simulink model "flightControlSystem"  (R2024a)
settings: Solver=ode3  StartTime=0  StopTime=TFinal  FixedStep=Ts  RelTol=1e-3  EnableMultiTasking=on
undefined symbols (not defined in the file or in its folder): BINARIZER_THRESHOLD, codertarget, COG_X, COG_Y, Controller, DiscIntNeverNeededParam, Discrete, DISK_KERNEL, Estimator, FLAG_WAIT_FOR_HOVERING, FOV, FRAME_SIZE_HEIGHT, FRAME_SIZE_WIDTH, g, G_B_GAIN, gray, init, MAX_RADIUS_CROWN, MIN_RADIUS_CROWN, orient_ref, pos_ref, Sensors, SQUARE_KERNEL, strel, Time, Ts, Vehicle, Z_HIGH, Z_LOW
libraries: simulink x35, sharedtransform x3, ctrlSharedLib x2, visionmorphops x2, sharedutil x1, parrotlib x1
(part 2 of 2)

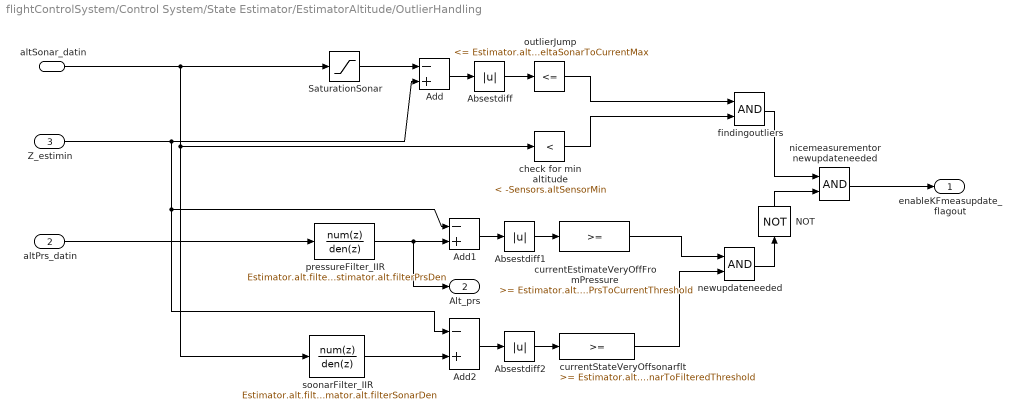
== system flightControlSystem/Control System/State Estimator/EstimatorAltitude/OutlierHandling ==
  altSonar_datin : Inport
  altPrs_datin : Inport  Port=2
  Z_estimin : Inport  Port=3
  Absestdiff : Abs  SaturateOnIntegerOverflow=off
  Absestdiff1 : Abs  SaturateOnIntegerOverflow=off
  Absestdiff2 : Abs  SaturateOnIntegerOverflow=off
  Add : Sum  Inputs=-+
  Add1 : Sum  Inputs=-+
  Add2 : Sum  Inputs=-+
  NOT : Logic  Operator=NOT  IconShape=distinctive  AllPortsSameDT=off  OutDataTypeStr=boolean
  SaturationSonar : Saturate  UpperLimit=-Sensors.altSensorMin  LowerLimit=-inf
  check for min altitude : simulink/Logic and Bit Operations/Compare To Constant  relop=<  const=-Sensors.altSensorMin  OutDataTypeStr=boolean
  currentEstimateVeryOffFromPressure : simulink/Logic and Bit Operations/Compare To Constant  relop=>=  const=Estimator.alt.deltaPrsToCurrentThreshold  OutDataTypeStr=boolean
  currentStateVeryOffsonarflt : simulink/Logic and Bit Operations/Compare To Constant  relop=>=  const=Estimator.alt.deltaSonarToFilteredThreshold  OutDataTypeStr=boolean
  findingoutliers : Logic  AllPortsSameDT=off  OutDataTypeStr=boolean
  newupdateneeded : Logic  AllPortsSameDT=off  OutDataTypeStr=boolean
  nicemeasurementor newupdateneeded : Logic  AllPortsSameDT=off  OutDataTypeStr=boolean
  outlierJump : simulink/Logic and Bit Operations/Compare To Constant  relop=<=  const=Estimator.alt.deltaSonarToCurrentMax  OutDataTypeStr=boolean
  pressureFilter_IIR : DiscreteFilter  Numerator=Estimator.alt.filterPrsNum  Denominator=Estimator.alt.filterPrsDen
  soonarFilter_IIR : DiscreteFilter  Numerator=Estimator.alt.filterSonarNum  Denominator=Estimator.alt.filterSonarDen
  enableKFmeasupdate_flagout : Outport  VectorParamsAs1DForOutWhenUnconnected=off
  Alt_prs : Outport  Port=2  VectorParamsAs1DForOutWhenUnconnected=off
  wires:
  Add1/1 -> Absestdiff1/1
  nicemeasurementor newupdateneeded/1 -> enableKFmeasupdate_flagout/1
  findingoutliers/1 -> nicemeasurementor newupdateneeded/1
  check for min altitude/1 -> findingoutliers/2
  outlierJump/1 -> findingoutliers/1
  SaturationSonar/1 -> Add/1
  Absestdiff/1 -> outlierJump/1
  Add/1 -> Absestdiff/1
  newupdateneeded/1 -> NOT/1
  Absestdiff2/1 -> currentStateVeryOffsonarflt/1
  altSonar_datin/1 -> SaturationSonar/1, soonarFilter_IIR/1, check for min altitude/1
  currentEstimateVeryOffFromPressure/1 -> newupdateneeded/1
  Z_estimin/1 -> Add1/1, Add2/1, Add/2
  Add2/1 -> Absestdiff2/1
  currentStateVeryOffsonarflt/1 -> newupdateneeded/2
  pressureFilter_IIR/1 -> Alt_prs/1, Add1/2
  altPrs_datin/1 -> pressureFilter_IIR/1
  soonarFilter_IIR/1 -> Add2/2
  Absestdiff1/1 -> currentEstimateVeryOffFromPressure/1
  NOT/1 -> nicemeasurementor newupdateneeded/2

== system flightControlSystem/Control System/State Estimator/EstimatorXYPosition/EstimatorVelocity ==
  opticalFlow_datin : Inport
  Z_estimin : Inport  Port=2  SampleTime=Ts
  sensorIMU_datin : Inport  Port=3
  orient_estimin : Inport  Port=4
  " " : Product  Inputs=**
  AccelerationHandling : Subsystem
  Compare To Constant : simulink/Logic and Bit Operations/Compare To Constant  relop=<  const=200*4  OutDataTypeStr=boolean
  Counter Free-Running : simulink/Sources/Counter Free-Running  NumBits=32  tsamp=-1
  DataHandling : Subsystem
  Delay : Delay  DelayLength=1  InitialCondition=0
  Gain : Gain  Gain=-1
  KalmanFilter_dxdy : ctrlSharedLib/Kalman Filter  TimeDomain=Discrete-Time  UseCurrentEstimator=on  ModelSource=Individual A, B, C, D matrices  ModelSourceVariable=ss(0.95,1,1,0,1)  A=eye(2)  B=Ts*eye(2)  C=eye(2)  D=0  NumberOfStates=1  NumberOfInputs=1  NumberOfOutputs=1  InitialEstimateSource=Dialog  X0=0  P0=10  UseK=off  UseGH=on  NumberOfProcessNoiseInputs=1  G=Estimator.pos.kfVelo.G  TimeInvariantG=on  H=Estimator.pos.kfVelo.H  TimeInvariantH=on  Q=Estimator.pos.kfVelo.Q  TimeInvariantQ=on  R=Estimator.pos.kfVelo.R  TimeInvariantR=on  N=Estimator.pos.kfVelo.N  TimeInvariantN=on  AddInputPort=on  AddEnablePort=on  OutputEstimatedY=off  OutputP=off  Ts=-1
  Select dxy : Selector  InputPortWidth=3  IndexOptions=Index vector (dialog)  Indices=[1 2]  OutputSizes=1
  Switch : Switch  Criteria=u2 > Threshold  SaturateOnIntegerOverflow=off  InputSameDT=off
  Z_estimin1 : InportShadow  Port=2  SampleTime=Ts
  opticalFlowErrorCorrect : Gain  Gain=1.15
  dxy_estimout : Outport  VectorParamsAs1DForOutWhenUnconnected=off
  wires:
  Delay/1 -> DataHandling/5(dxyOF_datin)
  Z_estimin/1 -> DataHandling/1(Z_estimin), AccelerationHandling/4(Z_estimin)
  KalmanFilter_dxdy/1 -> dxy_estimout/1, Delay/1
  sensorIMU_datin/1 -> AccelerationHandling/2(sensorIMU_datin), DataHandling/3(sensorIMU_datin)
  orient_estimin/1 -> AccelerationHandling/3(orient_estimin), DataHandling/2(orient_estimin)
  Select dxy/1 -> KalmanFilter_dxdy/2, AccelerationHandling/1(dxy_estimin), DataHandling/4(dxy_estimin)
  AccelerationHandling/1(acceleration_world) -> KalmanFilter_dxdy/1
  DataHandling/1(enable_flag) -> KalmanFilter_dxdy/3
  Switch/1 -> Select dxy/1
  " "/1 -> opticalFlowErrorCorrect/1
  Gain/1 -> " "/2
  opticalFlowErrorCorrect/1 -> Switch/3
  Compare To Constant/1 -> Switch/2
  opticalFlow_datin/1 -> " "/1, Switch/1
  Z_estimin1/1 -> Gain/1
  Counter Free-Running/1 -> Compare To Constant/1

== system flightControlSystem/Control System/State Estimator/EstimatorXYPosition/EstimatorXYPosition ==
  note: Switching from orientationControl to Position
      | control reset the current world position estimate
      | (happens when using no markers)
  dxy_estimin : Inport
  orient_estimin : Inport  Port=2  SampleTime=Ts
  controlModePosVSOrient_flagin : Inport  Port=3
  dz_estimin : Inport  Port=4
  Math Function : Math  Operator=transpose  SignedPower=on
  Mux2 : Mux  Inputs=2
  Product : Product  Multiplication=Matrix(*)
  Rotation Angles to Direction Cosine Matrix : sharedtransform/Rotation Angles to Direction Cosine Matrix  rotationOrder=ZYX  aMode=aMode
  SelectdXY : Selector  InputPortWidth=3  IndexOptions=Index vector (dialog)  Indices=[1 2]  OutputSizes=1
  SimplyIntegrateVelocity : DiscreteIntegrator  ExternalReset=rising  SampleTime=Ts  ICPrevOutput=DiscIntNeverNeededParam  ICPrevScaledInput=DiscIntNeverNeededParam
  XY_estimout : Outport  VectorParamsAs1DForOutWhenUnconnected=off
  wires:
  controlModePosVSOrient_flagin/1 -> SimplyIntegrateVelocity/2
  Product/1 -> SelectdXY/1
  Mux2/1 -> Product/2
  dz_estimin/1 -> Mux2/2
  SimplyIntegrateVelocity/1 -> XY_estimout/1
  dxy_estimin/1 -> Mux2/1
  orient_estimin/1 -> Rotation Angles to Direction Cosine Matrix/1
  Rotation Angles to Direction Cosine Matrix/1 -> Math Function/1
  SelectdXY/1 -> SimplyIntegrateVelocity/1
  Math Function/1 -> Product/1

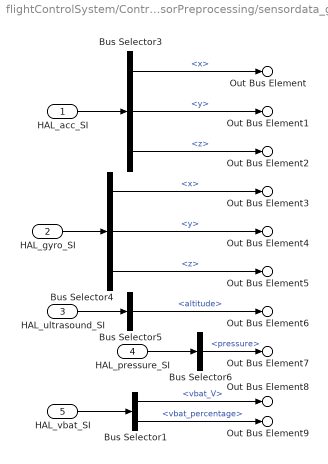
== system flightControlSystem/Control System/State Estimator/SensorPreprocessing/sensordata_group ==
  HAL_acc_SI : Inport  OutDataTypeStr=Bus: HAL_acc_SI_t
  HAL_gyro_SI : Inport  Port=2  OutDataTypeStr=Bus: HAL_gyro_SI_t
  HAL_ultrasound_SI : Inport  Port=3  OutDataTypeStr=Bus: HAL_ultrasound_SI_t
  HAL_pressure_SI : Inport  Port=4  OutDataTypeStr=Bus: HAL_pressure_SI_t
  HAL_vbat_SI : Inport  Port=5  OutDataTypeStr=Bus: HAL_vbat_SI_t
  Bus Selector1 : BusSelector  OutputSignals=vbat_V,vbat_percentage
  Bus Selector3 : BusSelector  OutputSignals=x,y,z
  Bus Selector4 : BusSelector  OutputSignals=x,y,z
  Bus Selector5 : BusSelector  OutputSignals=altitude
  Bus Selector6 : BusSelector  OutputSignals=pressure
  Out Bus Element : Outport  VectorParamsAs1DForOutWhenUnconnected=off  PortName=sensordata_datin  Element=ddx
  Out Bus Element1 : Outport  VectorParamsAs1DForOutWhenUnconnected=off  PortName=sensordata_datin  Element=ddy
  Out Bus Element2 : Outport  VectorParamsAs1DForOutWhenUnconnected=off  PortName=sensordata_datin  Element=ddz
  Out Bus Element3 : Outport  VectorParamsAs1DForOutWhenUnconnected=off  PortName=sensordata_datin  Element=p
  Out Bus Element4 : Outport  VectorParamsAs1DForOutWhenUnconnected=off  PortName=sensordata_datin  Element=q
  Out Bus Element5 : Outport  VectorParamsAs1DForOutWhenUnconnected=off  PortName=sensordata_datin  Element=r
  Out Bus Element6 : Outport  VectorParamsAs1DForOutWhenUnconnected=off  PortName=sensordata_datin  Element=altitude_sonar
  Out Bus Element7 : Outport  VectorParamsAs1DForOutWhenUnconnected=off  PortName=sensordata_datin  Element=prs
  Out Bus Element8 : Outport  VectorParamsAs1DForOutWhenUnconnected=off  PortName=sensordata_datin  Element=vbat_V
  Out Bus Element9 : Outport  VectorParamsAs1DForOutWhenUnconnected=off  PortName=sensordata_datin  Element=vbat_percentage
  wires:
  HAL_gyro_SI/1 -> Bus Selector4/1
  HAL_acc_SI/1 -> Bus Selector3/1
  HAL_pressure_SI/1 -> Bus Selector6/1
  HAL_ultrasound_SI/1 -> Bus Selector5/1
  Bus Selector4/1 -> Out Bus Element3/1  "<x>"
  Bus Selector3/3 -> Out Bus Element2/1  "<z>"
  Bus Selector4/3 -> Out Bus Element5/1  "<z>"
  Bus Selector5/1 -> Out Bus Element6/1  "<altitude>"
  Bus Selector6/1 -> Out Bus Element7/1  "<pressure>"
  Bus Selector4/2 -> Out Bus Element4/1  "<y>"
  Bus Selector3/1 -> Out Bus Element/1  "<x>"
  Bus Selector3/2 -> Out Bus Element1/1  "<y>"
  Bus Selector1/1 -> Out Bus Element8/1  "<vbat_V>"
  HAL_vbat_SI/1 -> Bus Selector1/1
  Bus Selector1/2 -> Out Bus Element9/1  "<vbat_percentage>"

== system flightControlSystem/Control System/State Estimator/EstimatorXYPosition/EstimatorVelocity/AccelerationHandling ==
  dxy_estimin : Inport
  sensorIMU_datin : Inport  Port=2
  orient_estimin : Inport  Port=3
  Z_estimin : Inport  Port=4
  Add : Sum  Inputs=-+
  Bus Selector1 : BusSelector  OutputSignals=ddx,ddy,ddz
  Deactivate Acceleration If OF is not used due to low altitude : simulink/Logic and Bit Operations/Compare To Constant  relop=<=  const=Estimator.pos.opticalFlowZMax  OutDataTypeStr=boolean
  Logical Operator : Logic  Operator=OR  AllPortsSameDT=off  OutDataTypeStr=boolean
  Mux6 : Mux  Inputs=3
  Product : Product  Inputs=3
  Product1 : Product  Multiplication=Matrix(*)
  Rotation Angles to Direction Cosine Matrix : sharedtransform/Rotation Angles to Direction Cosine Matrix  rotationOrder=ZYX  aMode=aMode
  SelectPlanarddxy : Selector  InputPortWidth=3  IndexOptions=Index vector (dialog)  Indices=[1 2]  OutputSizes=1
  Selector : Selector  InputPortWidth=2  IndexOptions=Index vector (dialog)  Indices=1  OutputSizes=1
  Selector1 : Selector  InputPortWidth=2  IndexOptions=Index vector (dialog)  Indices=2  OutputSizes=1
  do not use acc if optical flow never available (Note OF@60Hz but ZOH to 200!) : simulink/Logic and Bit Operations/Compare To Constant  relop=~=  const=0  OutDataTypeStr=boolean
  do not use acc if optical flow never available (Note OF@60Hz but ZOH to 200!)1 : simulink/Logic and Bit Operations/Compare To Constant  relop=~=  const=0  OutDataTypeStr=boolean
  gainaccinput : Gain  Gain=Estimator.pos.accelerationInputGain  OutDataTypeStr=single
  gravity : Constant  Value=[0 0 -g]
  acceleration_world : Outport  OutDataTypeStr=single  VectorParamsAs1DForOutWhenUnconnected=off
  wires:
  do not use acc if optical flow never available (Note OF@60Hz but ZOH to 200!)1/1 -> Logical Operator/2
  do not use acc if optical flow never available (Note OF@60Hz but ZOH to 200!)/1 -> Logical Operator/1
  Logical Operator/1 -> Product/1
  Selector1/1 -> do not use acc if optical flow never available (Note OF@60Hz but ZOH to 200!)1/1
  Selector/1 -> do not use acc if optical flow never available (Note OF@60Hz but ZOH to 200!)/1
  dxy_estimin/1 -> Selector1/1, Selector/1
  Product/1 -> acceleration_world/1
  Deactivate Acceleration If OF is not used due to low altitude/1 -> Product/3
  Z_estimin/1 -> Deactivate Acceleration If OF is not used due to low altitude/1
  Add/1 -> SelectPlanarddxy/1
  Product1/1 -> Add/1
  gravity/1 -> Product1/2
  gainaccinput/1 -> Product/2
  SelectPlanarddxy/1 -> gainaccinput/1
  Bus Selector1/3 -> Mux6/3  "<ddz>"
  Bus Selector1/1 -> Mux6/1  "<ddx>"
  sensorIMU_datin/1 -> Bus Selector1/1
  Mux6/1 -> Add/2
  Bus Selector1/2 -> Mux6/2  "<ddy>"
  orient_estimin/1 -> Rotation Angles to Direction Cosine Matrix/1
  Rotation Angles to Direction Cosine Matrix/1 -> Product1/1

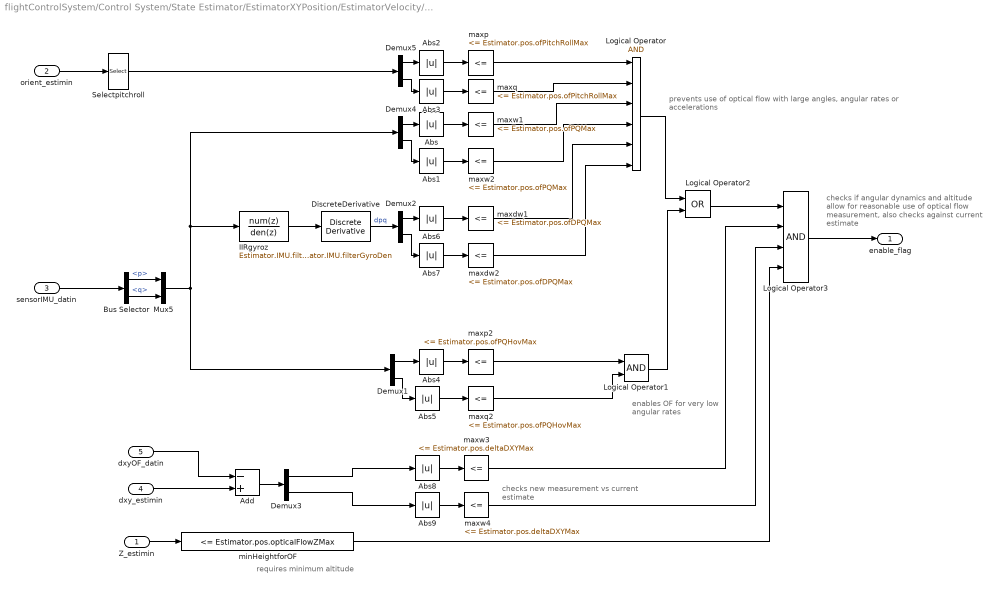
== system flightControlSystem/Control System/State Estimator/EstimatorXYPosition/EstimatorVelocity/DataHandling ==
  note: prevents use of optical flow with large angles, angular rates or accelerations
  note: enables OF for very
      | low angular rates
  note: checks if angular dynamics and altitude allow for
      | reasonable use of optical flow measurement,
      | also checks against current estimate
  note: checks new measurement vs current estimate
  note: requires minimum altitude
  Z_estimin : Inport
  orient_estimin : Inport  Port=2
  sensorIMU_datin : Inport  Port=3
  dxy_estimin : Inport  Port=4
  dxyOF_datin : Inport  Port=5
  Abs{,1..9} (10 alike) : Abs  SaturateOnIntegerOverflow=off
  Add : Sum  Inputs=-+
  Bus Selector : BusSelector  OutputSignals=p,q
  Demux{1..5} (5 alike) : Demux  Outputs=2
  DiscreteDerivative : simulink/Discrete/Discrete Derivative  gainval=1.0  ICPrevScaledInput=0.0  OutMin=[]  OutMax=[]  OutDataType=fixdt(1, 16)  OutScaling=2^-10  DoSatur=off
  IIRgyroz : DiscreteFilter  Numerator=Estimator.IMU.filterGyroNum  Denominator=Estimator.IMU.filterGyroDen
  Logical Operator : Logic  Inputs=6  AllPortsSameDT=off  OutDataTypeStr=boolean
  Logical Operator1 : Logic  AllPortsSameDT=off  OutDataTypeStr=boolean
  Logical Operator2 : Logic  Operator=OR  AllPortsSameDT=off  OutDataTypeStr=boolean
  Logical Operator3 : Logic  Inputs=4  AllPortsSameDT=off  OutDataTypeStr=boolean
  Mux5 : Mux  Inputs=2
  Selectpitchroll : Selector  InputPortWidth=3  IndexOptions=Index vector (dialog)  Indices=[2 3]  OutputSizes=1
  maxdw1 : simulink/Logic and Bit Operations/Compare To Constant  relop=<=  const=Estimator.pos.ofDPQMax  OutDataTypeStr=boolean
  maxdw2 : simulink/Logic and Bit Operations/Compare To Constant  relop=<=  const=Estimator.pos.ofDPQMax  OutDataTypeStr=boolean
  maxp : simulink/Logic and Bit Operations/Compare To Constant  relop=<=  const=Estimator.pos.ofPitchRollMax  OutDataTypeStr=boolean
  maxp2 : simulink/Logic and Bit Operations/Compare To Constant  relop=<=  const=Estimator.pos.ofPQHovMax  OutDataTypeStr=boolean
  maxq : simulink/Logic and Bit Operations/Compare To Constant  relop=<=  const=Estimator.pos.ofPitchRollMax  OutDataTypeStr=boolean
  maxq2 : simulink/Logic and Bit Operations/Compare To Constant  relop=<=  const=Estimator.pos.ofPQHovMax  OutDataTypeStr=boolean
  maxw1 : simulink/Logic and Bit Operations/Compare To Constant  relop=<=  const=Estimator.pos.ofPQMax  OutDataTypeStr=boolean
  maxw2 : simulink/Logic and Bit Operations/Compare To Constant  relop=<=  const=Estimator.pos.ofPQMax  OutDataTypeStr=boolean
  maxw3 : simulink/Logic and Bit Operations/Compare To Constant  relop=<=  const=Estimator.pos.deltaDXYMax  OutDataTypeStr=boolean
  maxw4 : simulink/Logic and Bit Operations/Compare To Constant  relop=<=  const=Estimator.pos.deltaDXYMax  OutDataTypeStr=boolean
  minHeightforOF : simulink/Logic and Bit Operations/Compare To Constant  relop=<=  const=Estimator.pos.opticalFlowZMax  OutDataTypeStr=boolean
  enable_flag : Outport  VectorParamsAs1DForOutWhenUnconnected=off
  wires:
  minHeightforOF/1 -> Logical Operator3/4
  IIRgyroz/1 -> DiscreteDerivative/1
  Mux5/1 -> Demux1/1, IIRgyroz/1, Demux4/1
  maxw4/1 -> Logical Operator3/3
  maxw3/1 -> Logical Operator3/2
  dxyOF_datin/1 -> Add/1
  Demux3/2 -> Abs9/1
  Demux3/1 -> Abs8/1
  dxy_estimin/1 -> Add/2
  Add/1 -> Demux3/1
  Abs9/1 -> maxw4/1
  Abs8/1 -> maxw3/1
  Logical Operator2/1 -> Logical Operator3/1
  Logical Operator3/1 -> enable_flag/1
  DiscreteDerivative/1 -> Demux2/1  "dpq"
  Demux2/2 -> Abs7/1
  Demux2/1 -> Abs6/1
  Abs7/1 -> maxdw2/1
  Abs6/1 -> maxdw1/1
  Logical Operator1/1 -> Logical Operator2/2
  Demux1/2 -> Abs5/1
  Demux1/1 -> Abs4/1
  Abs5/1 -> maxq2/1
  Abs4/1 -> maxp2/1
  Abs3/1 -> maxq/1
  Abs2/1 -> maxp/1
  Demux4/2 -> Abs1/1
  Demux4/1 -> Abs/1
  Abs1/1 -> maxw2/1
  Abs/1 -> maxw1/1
  Z_estimin/1 -> minHeightforOF/1
  Logical Operator/1 -> Logical Operator2/1
  maxw1/1 -> Logical Operator/3
  Bus Selector/1 -> Mux5/1  "<p>"
  Selectpitchroll/1 -> Demux5/1
  sensorIMU_datin/1 -> Bus Selector/1
  maxq2/1 -> Logical Operator1/2
  Bus Selector/2 -> Mux5/2  "<q>"
  maxp/1 -> Logical Operator/1
  maxw2/1 -> Logical Operator/4
  orient_estimin/1 -> Selectpitchroll/1
  maxdw1/1 -> Logical Operator/5
  maxdw2/1 -> Logical Operator/6
  maxq/1 -> Logical Operator/2
  Demux5/1 -> Abs2/1
  Demux5/2 -> Abs3/1
  maxp2/1 -> Logical Operator1/1

== stateflow chart flightControlSystem/Image Processing System/Waypoints Follower/state machine ==
  state STATE [group]
    - ON_TRACK: the Image Processing System detects the lane. The drone is on the lane.
    - END_TRACK: it indicates the end of the lane.
  state OUTPUT [group]
    - FLAG: it indicates the presence or not of the track path
  state INPUT [group]
    - FLAG_TRACK: flag raises when the track is detected from Image Processing System.
  state END_TRACK
    entry: flag=0;
  state ON_TRACK
    entry: flag=1;
  state TAKE_OFF
    entry: flag=1;
  ON_TRACK -> END_TRACK : [flag_track==0]
  TAKE_OFF -> ON_TRACK : [flag_track==1]
  (default) -> TAKE_OFF
  data: flag_track input; flag output

== matlab function flightControlSystem/Image Processing System/Image Binarization ==
  data: r input; binarized_frame output; g input; b input; G_B_GAIN parameter; BINARIZER_THRESHOLD parameter
function binarized_frame = binarizer(r, g, b, G_B_GAIN, BINARIZER_THRESHOLD)
% The MATLAB function computes a binarized frame starting from a frame 
% expressed in the RGB file format. 
%
% Inputs:
% - r: Red channel frame
% - g: Green channel frame
% - b: Blue channel frame
%
% Output:
% - binarize_frame: the binarized frame
%
% Parameters:
% - G_B_GAIN: used to reduce the amount of green and blue colors inside the frame
% - BINARIZER_THRESHOLD: threshold to detect only the track inside the frame 

frame= r - (g/G_B_GAIN) - (b/G_B_GAIN);

binarized_frame = frame >= BINARIZER_THRESHOLD;

end

== matlab function flightControlSystem/Control System/Path Planning/MPC block ==
  data: x_err input; roll_ref output; y_err input; phi input; theta input; psi input; vx input; vy input; vz input; p input; q input; r input; takeoff_flag input; pitch_ref output; yaw_ref output; thrust output; x_est input; y_est input
function [roll_ref, pitch_ref, yaw_ref, thrust] = fcn( ...
        x_err, y_err, phi, theta, psi, ...
        vx, vy, vz, p, q, r, takeoff_flag, x_est, y_est)
%#codegen
% POSITION MODE: outputs carry [x_planned; y_planned; z_planned] (pos_ref).
% Output port names kept as roll/pitch/yaw_ref only to preserve the Mux wiring.
[roll_ref, pitch_ref, yaw_ref, thrust] = mpc_racing_controller( ...
    x_err, y_err, phi, theta, psi, ...
    vx, vy, vz, p, q, r, takeoff_flag, x_est, y_est);
end

== matlab function flightControlSystem/Control System/Path Planning/Take off Checker ==
  data: flag_activate_PP output; z_est input; Z_LOW parameter; Z_HIGH parameter; FLAG_WAIT_FOR_HOVERING parameter
function flag_activate_PP = height_checker(z_est, Z_LOW, Z_HIGH, FLAG_WAIT_FOR_HOVERING)
% This MATLAB function raise a flag when the drone is hovering by using the
% z_low and z_high variable which are threshold level expressed in meters. The output is a
% flag that permits the path planner to be activated and perform the
% trajectory tracking.
%
% Inputs:
% - z_low: low threshold height, in meters
% - z_high: high threshold height, in meters
% - z_est: estimation of drone's height 
% - FLAG_WAIT_FOR_HOVERING: the flag is used to decide if path planner is
% activie before or after drone takes off (TRUE/FALSE)
%
% Output:
% - flag_activate_PP: the flag is used to activate the Path Planner.

if FLAG_WAIT_FOR_HOVERING == 0
    
    if z_est < Z_LOW && z_est > Z_HIGH
        
        flag_activate_PP = 1 ;
    else
        
        flag_activate_PP = 0 ;
        
    end
    
else
    
    flag_activate_PP = 1 ;
    
end

end

== matlab function flightControlSystem/Control System/Path Planning/MATLAB Function ==
  data: x_err_tr input; x_error output; y_err_tr input; x_err_ea input; y_err_ea input; flag_ea input; flag_ho input; y_error output
function [x_error, y_error] = decision_making(x_err_tr, y_err_tr, x_err_ea, ...
    y_err_ea, flag_ea, flag_ho)
% The MALTAB function sends the error along x- and y-axis to the drone 
% trajectory controller. When the "flag_ea" is low, the position errors
% are computed as the difference between the end-marker and the drone
% CoG. Instead, when the flag is high, the errors are computed by the
% Image Processing System.
%
% Inputs:
% - x_err_tr: tracking error along the x-axis. The error is expressed in 
% pixels.
% - y_err_tr: tracking error along the y-axis. The error is expressed in 
% pixels.
% - x_err_ea: position error along the x-axis when the end-marker is 
% detected. The error is expressed in pixels.
% - y_err_ea: position error along the y-axis when the end-marker is
% detected. The error is expressed in pixels.
% - flag_ea: the flag allows to check if the end-maker is recognized.
% - flag_ho: the flag allows to check if the drone is able to fly.
%   
% Outputs
% - x_error: error between the drone CoG and the track/end-marker along the 
% x-axis. The error is expressed in pixels.
% - y_error: error between the drone CoG and the track/end-marker along the
% y-axis. The error is expressed in pixels

if flag_ho == 1
    
    if flag_ea == 0
        
        x_error=x_err_tr;
        y_error=y_err_tr;
              
    else
        
        x_error=x_err_ea;
        y_error=y_err_ea;
        
    end
    
else
    
    x_error=0;
    y_error=0;
    
end
    
end

== matlab function flightControlSystem/Image Processing System/Waypoints Follower/waypoints 1 ==
  data: frame input; error_y_track output; error_x_track output; x_ref_prev input; y_ref_prev input; orientation_track output; flag_track output; flag_track_prev input; MIN_RADIUS_CROWN parameter; MAX_RADIUS_CROWN parameter; FOV parameter; COG_X parameter; COG_Y parameter
function [error_y_track, error_x_track, orientation_track, flag_track] = ...
error_pixel_generator(frame, x_ref_prev, y_ref_prev, flag_track_prev, ...
MIN_RADIUS_CROWN, MAX_RADIUS_CROWN, FOV, COG_X, COG_Y)
% LINE-TRACING detector (connected + predictive).
%
% Instead of "pick an arm by angle", it MARCHES along the connected line:
% starting at the drone centre, heading = the previous lane direction, it steps
% forward and at each step snaps to the local line and rotates its heading to
% follow the line's curve.  Because it walks ALONG one connected line:
%   - it never jumps to a different (disconnected) arm  -> no fork flipping
%   - it follows the line wherever it bends, incl. backward (the heading rotates
%     with the line; only a near-full reversal > TURN_MAX is blocked)
% The "lock" persists through the model feedback (orientation_track comes from
% the previous output via the z^-1 blocks).  I/O identical to the block.
%
% paste over the whole "waypoints 1" block body.

%#codegen

% ── parameters ────────────────────────────────────────────────────────────
STEP_LEN = 2.0;    % march step length [px]
N_STEP   = 12;     % number of steps  (look-ahead ~= STEP_LEN*N_STEP px)
WIN_R    = 15;      % search half-window around each step [px]
TURN_MAX = 2.6;   % rad ~135deg : max turn per step (blocks only the ~back)
DIR_LP   = 0.20;    % heading low-pass per step (1 = snap hard to local line)

% lane heading from the previous tracking point (= march seed, and an output)
orientation_track = atan2(-x_ref_prev, y_ref_prev);
orientation_track = mod(orientation_track, 2*pi);

imax = size(frame,1);
jmax = size(frame,2);
error_x_track = 0;
error_y_track = 0;
flag_track    = false;

if flag_track_prev == 0
    % ── INITIAL acquisition: plain crown-ring centroid (detect line @ takeoff)
    sumi = 0.0; sumj = 0.0; cnt = 0.0;
    for i = (COG_X-MAX_RADIUS_CROWN):(COG_X+MAX_RADIUS_CROWN)
        for j = (COG_Y-MAX_RADIUS_CROWN):(COG_Y+MAX_RADIUS_CROWN)
            if i>=1 && i<=imax && j>=1 && j<=jmax
                nrm = sqrt((i-(COG_X-0.5))^2 + (j-(COG_Y-0.5))^2);
                if nrm>=MIN_RADIUS_CROWN && nrm<=MAX_RADIUS_CROWN && frame(i,j)==1
                    sumi = sumi+i; sumj = sumj+j; cnt = cnt+1.0;
                end
            end
        end
    end
    if cnt > 0.0
        error_x_track = -(round(sumi/cnt) - COG_X);
        error_y_track =  (round(sumj/cnt) - COG_Y);
        flag_track    = true;
    end

else
    % ── MARCH along the connected line ────────────────────────────────────
    ci   = COG_X - 0.5;          % current march position (row, col)
    cj   = COG_Y - 0.5;
    mdir = orientation_track;    % start heading = previous lane direction
    nf   = 0.0;

    for s = 1:N_STEP
        % candidate point one step ahead along the current heading
        ti = ci + STEP_LEN*sin(mdir);
        tj = cj + STEP_LEN*cos(mdir);
        % centroid of line pixels in the window that lie in the forward cone
        sumi = 0.0; sumj = 0.0; cnt = 0.0;
        for ii = floor(ti-WIN_R):ceil(ti+WIN_R)
            for jj = floor(tj-WIN_R):ceil(tj+WIN_R)
                if ii>=1 && ii<=imax && jj>=1 && jj<=jmax && frame(ii,jj)==1
                    ang = atan2(ii-ci, jj-cj);                 % current pos -> pixel
                    dev = abs(atan2(sin(ang-mdir), cos(ang-mdir)));
                    if dev <= TURN_MAX
                        sumi = sumi+ii; sumj = sumj+jj; cnt = cnt+1.0;
                    end
                end
            end
        end
        if cnt < 1.0
            break;                          % line ended ahead -> stop
        end
        ni = sumi/cnt; nj = sumj/cnt;        % local line centre
        nd = atan2(ni-ci, nj-cj);            % heading toward it
        mdir = mdir + DIR_LP*atan2(sin(nd-mdir), cos(nd-mdir));   % rotate to follow
        ci = ni; cj = nj;                    % advance along the line
        nf = nf + 1.0;
    end

    if nf > 0.0
        error_x_track = -(round(ci) - COG_X);
        error_y_track =  (round(cj) - COG_Y);
        flag_track    = true;
    end
end

end

== matlab function flightControlSystem/Image Processing System/Land Mark Detector ==
  data: output output; binary input; waypoint_follower_variable input; FRAME_SIZE_WIDTH parameter; FRAME_SIZE_HEIGHT parameter; COG_Y parameter; COG_X parameter
function output = end_marker_detector(binary, waypoint_follower_variable, ...
    FRAME_SIZE_WIDTH, FRAME_SIZE_HEIGHT, COG_Y, COG_X)
% The MATLAB function computes the errors along the x- and y-axis between
% the drone COG and the middle of the lane. The end marker is detected by 
% using a disk kernel. This function is active only when the drone has 
% arrived at the end of the path.
%
%
% Inputs:
% - binary: binarized frame obtained as the convolution with a disk kernel
% - x_ref_prev: previous value of the tracking point along the x-axis of 
% the track line. It is used as a reference for tracking the path.
% - y_ref_prev: previous value of the tracking point along the y-axis of 
% the track line. It is used as a reference for tracking the path. 
% - flag_track_prev: previous value assumed by the flag variablle, i.e., 
% the previous state of the drone (over the track / not over the track).
%
%
% Outputs:
% - error_y_end_marker: error between the CoG of the drone and a point of the 
% lane in the forward direction along the y-axis. It is expressed in
% pixels.
% - error_x_end_maker: error between the CoG of the drone and a point of the 
% lane in the forward direction along the x-axis. It is expressed in pixels. 
% - flag_end_marker: it is TURE if the Image Processing System detects 
% the end marker.
% - yaw: heading angle of the lane in the image plane.
%
%
%Parameters:
% - COG_X: position of the drone CoG along x-axis of the reference frame.
% - COG_Y: position of the drone CoG along y-axis of the reference frame.
% - FRAME_SIZE_WIDTH: width of the frame.
% - FRAME_SIZE_HEIGHT: height of the frame.

persistent column_accumulator
persistent count_pixel
persistent row_accumulator

if isempty(column_accumulator)
    column_accumulator = 0;
end

if isempty(count_pixel)
    count_pixel = 0;
end

if isempty(row_accumulator)
    row_accumulator = 0;
end

flag_track = waypoint_follower_variable(3);


% check if the track is ended
if ~flag_track

    for i=1:FRAME_SIZE_HEIGHT

        for j=1:FRAME_SIZE_WIDTH

            %check all the pixel belonging to the end marker
            if binary(i,j)==1
                count_pixel = count_pixel +1;
                column_accumulator = column_accumulator + j;
                row_accumulator = row_accumulator + i;

            end

        end
    end
    
    if count_pixel ~= 0
        flag_end_marker=1;
        center_x = round(row_accumulator/count_pixel);
        center_y = round(column_accumulator/count_pixel);
    else
        flag_end_marker=0;
        center_x=1;
        center_y=1;
    end

else
    
    center_x = 0;
    center_y = 0;
    flag_end_marker = 0;

end

% Calculate the medium point of the end marker
error_x_end_marker = -(center_x - COG_X);
error_y_end_marker = (center_y - COG_Y);

% reset of the persistent variables
count_pixel = 0;
column_accumulator = 0;
row_accumulator = 0;

output = [error_x_end_marker, error_y_end_marker, flag_end_marker];

end
